simulink model "sinfcn"  (R2021a)
settings: Solver=VariableStepAuto  StartTime=0.0  StopTime=0.005  RelTol=1e-3
undefined symbols (not defined in the file): C1, C2, R1, R2, Vs
settings Model: Creator=spbro  LastModifiedBy=spbro

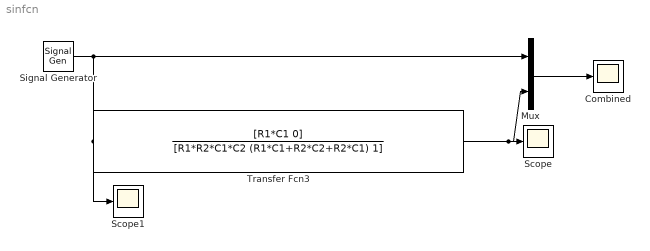
== system sinfcn ==
  Combined : Scope
  Mux : Mux  Inputs=2
  Scope : Scope
  Scope1 : Scope
  Signal Generator : SignalGenerator  Amplitude=Vs  Frequency=500
  Transfer Fcn3 : TransferFcn  Numerator=[R1*C1 0]  Denominator=[R1*R2*C1*C2 (R1*C1+R2*C2+R2*C1) 1]
  wires:
  Mux/1 -> Combined/1
  Signal Generator/1 -> Scope1/1, Transfer Fcn3/1, Mux/1
  Transfer Fcn3/1 -> Mux/2, Scope/1
